simulink model "AllObserverComparisonTest1_08"  (R2019b)
settings: Solver=ode4  StartTime=0.0  StopTime=timeStop  FixedStep=timeStep  RelTol=1e-3
values from neighbouring files (symbols this model uses):
  focalLen = 20    [paraSetting.m]
  k81 = 30    [paraSetting.m]
  k82 = 30    [paraSetting.m]
  k83 = 3.6    [paraSetting.m]
settings Model: PauseTimes=1.3  Creator=lixiangfei  LastModifiedBy=lixiangfei
settings DataIOCC: ReturnWorkspaceOutputs=off
settings DebuggingCC: ArithmeticOperatorsInVariantConditions=warning
settings SFSimCC: SimUseLocalCustomCode=off  CustomCodeUndefinedFunction=UseInterfaceOnly
settings RTWCC: RTWUseLocalCustomCode=off

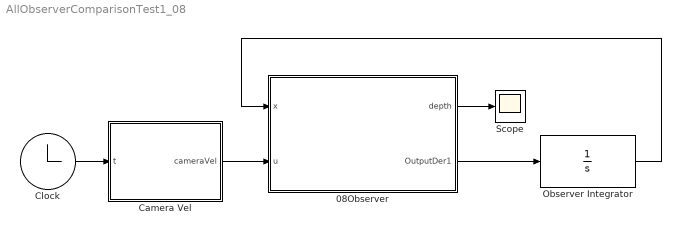
== system AllObserverComparisonTest1_08 ==
  08Observer : MATLAB Function  TreatAsAtomicUnit=on
  Camera Vel : MATLAB Function  TreatAsAtomicUnit=on
  Clock : Clock
      settings: Decimation=5
  Observer Integrator : Integrator  InitialCondition=[3, 1.5, 0.25, 1200, 1000, 25]
  Scope : Scope
  wires:
  Clock/1 -> Camera Vel/1(t)
  08Observer/2(OutputDer1) -> Observer Integrator/1
  Observer Integrator/1 -> 08Observer/1(x)
  Camera Vel/1(cameraVel) -> 08Observer/2(u)
  08Observer/1(depth) -> Scope/1

== matlab function AllObserverComparisonTest1_08/Camera Vel ==
  data: t input; cameraVel output; modelSelection parameter
function cameraVel = Model(t, modelSelection)
%% 设定如下透视系统模型，模型为 Xdot = AX + B
cameraVel = zeros(1,6);

if modelSelection == 1
% 测试1.该模型用于验证观测器的收敛性,是否收敛于任意大的初值
    cameraVel(1) = 0.1;
    cameraVel(2) = 0.2;
    cameraVel(3) = -0.8;
    cameraVel(4) = sin(pi*t);
    cameraVel(5) = pi/15;
    cameraVel(6) = pi/8; 
end
end

== matlab function AllObserverComparisonTest1_08/08Observer ==
  settings: updateMethod=DISCRETE
  data: depth output; x input; u input; OutputDer1 output; focalLen parameter; k81 parameter; k82 parameter; k83 parameter
function [depth,OutputDer1] = Observer(x, u, focalLen, k81, k82, k83)
%% 模型初始化
% 初始化输出
OutputDer1 = zeros(1,6);
depth = zeros(1,2);

% 系统动力学
OutputDer1(1:3) = [-focalLen*x(3), 0, x(1)*x(3), x(1)*x(2)/focalLen, -(focalLen+x(1)^2/focalLen), x(2);
          0, -focalLen*x(3), x(2)*x(3), (focalLen+x(2)^2/focalLen), -x(1)*x(2)/focalLen, -x(1);
          0, 0, x(3)^2, x(2)*x(3)/focalLen, -x(1)*x(3)/focalLen, 0] * u';
      
%% Feature Depth Observation for Image-based Visual Servoing: Theory and Experiments
% 2008 IJRR; Author:  Alessandro De Luca et al.
% 观测误差
e81 = x(1) - x(4);
e82 = x(2) - x(5);

% 系统输出, 未加噪声
y8 = [x(4), x(5)]';

OutputDer1(4:6) = [-focalLen*x(6), 0, y8(1)*x(6), y8(1)*y8(2)/focalLen, -(focalLen+y8(1)^2/focalLen), y8(2);
          0, -focalLen*x(6), y8(2)*x(6), (focalLen+y8(2)^2/focalLen), -y8(1)*y8(2)/focalLen, -y8(1);
          0, 0, x(6)^2, y8(2)*x(6)/focalLen, -y8(1)*x(6)/focalLen, 0] * u' + ...
          [k81*e81, k82*e82, k83*((-focalLen*u(1)+y8(1)*u(3))*e81+((-focalLen*u(2)+y8(2)*u(3))*e82))]';
      
%% 输出深度值
% 模型的真实值
state = x;
depth(1) = 1/state(3);

% Feature Depth Observation for Image-based Visual Servoing: Theory and Experiments
depth(2) = 1/state(6);
end
